simulink model "Linearized_FullorderObserver"  (R2020b)
settings: Solver=VariableStepAuto  StartTime=0.0  StopTime=10  RelTol=1e-3
undefined symbols (not defined in the file): A, B, C, K_trackink_1, K_trackink_2, LFobserver
settings Model: Creator=YSN  LastModifiedBy=YSN

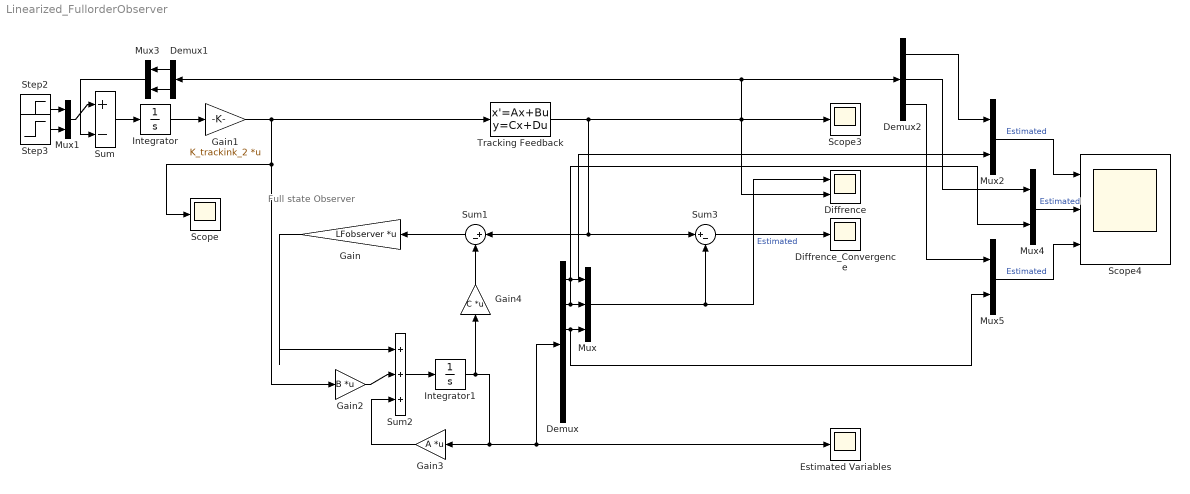
== system Linearized_FullorderObserver ==
  note: Full state Observer
  Demux : Demux  Outputs=6
  Demux1 : Demux  Outputs=3
  Demux2 : Demux  Outputs=3
  Diffrence : Scope  NumInputPorts=2
  Diffrence_Convergence : Scope
  Estimated Variables : Scope
  Gain : Gain  Gain=LFobserver  Multiplication=Matrix(K*u)
  Gain1 : Gain  Gain=K_trackink_2  Multiplication=Matrix(K*u)
  Gain2 : Gain  Gain=B  Multiplication=Matrix(K*u)
  Gain3 : Gain  Gain=A  Multiplication=Matrix(K*u)
  Gain4 : Gain  Gain=C  Multiplication=Matrix(K*u)
  Integrator : Integrator
  Integrator1 : Integrator
  Mux : Mux  Inputs=3
  Mux{1..5} (5 alike) : Mux  Inputs=2
  Scope : Scope
  Scope3 : Scope
  Scope4 : Scope  NumInputPorts=3
  Step2 : Step  Time=100  SampleTime=0
  Step3 : Step  Time=100  SampleTime=0
  Sum : Sum  Inputs=|+-
  Sum1 : Sum  Inputs=|+-
  Sum2 : Sum  Inputs=|+++
  Sum3 : Sum  Inputs=|+-
  Tracking Feedback : StateSpace  A=A-B*K_trackink_1  B=B  C=C  D=[0 0;0 0;0 0]  InitialCondition=[0.1 0.1 -0.1 0 0 0]  ContinuousStateAttributes='Helicopter'
  wires:
  Sum/1 -> Integrator/1
  Integrator/1 -> Gain1/1
  Step3/1 -> Mux1/2
  Mux1/1 -> Sum/1
  Demux1/1 -> Mux3/1
  Demux1/3 -> Mux3/2
  Mux3/1 -> Sum/2
  Step2/1 -> Mux1/1
  Sum3/1 -> Diffrence_Convergence/1
  Mux/1 -> Diffrence/1, Sum3/2  "Estimated"
  Integrator1/1 -> Demux/1, Estimated Variables/1, Gain3/1, Gain4/1
  Gain1/1 -> Scope/1, Gain2/1, Tracking Feedback/1
  Sum1/1 -> Gain/1
  Gain2/1 -> Sum2/2
  Demux/3 -> Mux5/2, Mux/3
  Gain/1 -> Sum2/1
  Gain4/1 -> Sum1/2
  Demux/2 -> Mux4/2, Mux/2
  Sum2/1 -> Integrator1/1
  Gain3/1 -> Sum2/3
  Tracking Feedback/1 -> Sum3/1, Sum1/1, Diffrence/2, Demux2/1, Demux1/1, Scope3/1
  Demux/1 -> Mux2/2, Mux/1
  Demux2/1 -> Mux2/1
  Demux2/2 -> Mux4/1
  Demux2/3 -> Mux5/1
  Mux2/1 -> Scope4/1  "Estimated"
  Mux4/1 -> Scope4/2  "Estimated"
  Mux5/1 -> Scope4/3  "Estimated"
